simulink library "PhD_Library"  (R2018a)
settings: Solver=VariableStepAuto  StartTime=0.0  StopTime=10.0  RelTol=1e-3
values from neighbouring files (symbols this model uses):
  Ts = Ts_c    (= 1e-07)    [PlantStateEquations_abc_Script.m]
undefined symbols (not defined in the file or in its folder): D1, Delta, DiscIntNeverNeededParam, ESS, f_LPF_noise, fcutouti, fcutoutv, fn, fsw, Iap, Kp, PCC, Sn, tctrl, Ti, Ts_control, Ts_PWM, Uabp, Uanp, WT, X, zeta
libraries: $bdroot x84, powerlib_meascontrol x59, powerlib x56, peTransforms x32, cstblocks x2, simulink x2
(part 3 of 5)

== system PhD_Library/Offshore_Oil_and_Wind/LSC_LCL_Trafo_NoSwitching ==
  Open_Close_Breaker : Inport
  Vabcref : Inport  Port=2
  Bus Creator : BusCreator  Inputs=6
  Controlled Voltage Source : powerlib/Electrical Sources/Controlled Voltage Source  Initialize=on  Source_Type=AC  Amplitude=Uab*(2/3)^0.5  Phase=30  Frequency=fn  Measurements=None
  Controlled Voltage Source1 : powerlib/Electrical Sources/Controlled Voltage Source  Initialize=on  Source_Type=AC  Amplitude=Uab*(2/3)^0.5  Phase=30-120  Frequency=fn  Measurements=None
  Controlled Voltage Source2 : powerlib/Electrical Sources/Controlled Voltage Source  Initialize=on  Source_Type=AC  Amplitude=Uab*(2/3)^0.5  Phase=30+120  Frequency=fn  Measurements=None
  Demux2 : Demux  Outputs=3
  HV : powerlib/Measurements/Three-Phase V-I Measurement  VoltageMeasurement=phase-to-ground  SetLabelV=off  LabelV=vgrid  Vpu=off  VpuLL=off  CurrentMeasurement=yes  SetLabelI=off  LabelI=igrid  Ipu=off  Pbase=sn  Vbase=uab  OutputType=Complex  PhasorSimulation=off  PSBequivalent=0
  High Res Grounding : powerlib/Elements/Three-Phase Parallel RLC Load  LConnTagsString=A|B|C  Configuration=Y (grounded)  NominalVoltage=Uab  Vabc=[1e3 1e3 1e3]  Vabcp=[1e3 1e3 1e3]  NominalFrequency=fn  UnbalancedPower=off  ActivePower=0.001  InductivePower=0  CapacitivePower=0  Pabc=[10e3 9e3 11e3]  QLabc=[100 90 110]  QCabc=[100 90 110]  Pabcp=[10e3 9e3 11e3]  QLabcp=[100 90 110]  QCabcp=[100 90 110]  Measurements=None  LoadType=constant Z
  INV : powerlib/Measurements/Three-Phase V-I Measurement  VoltageMeasurement=phase-to-ground  SetLabelV=off  LabelV=vconv  Vpu=off  VpuLL=off  CurrentMeasurement=yes  SetLabelI=off  LabelI=iconv  Ipu=off  Pbase=sn  Vbase=uab  OutputType=Complex  PhasorSimulation=off  PSBequivalent=0
  LV : powerlib/Measurements/Three-Phase V-I Measurement  VoltageMeasurement=phase-to-ground  SetLabelV=off  LabelV=vgrid  Vpu=off  VpuLL=off  CurrentMeasurement=yes  SetLabelI=off  LabelI=igrid  Ipu=off  Pbase=sn  Vbase=uab  OutputType=Complex  PhasorSimulation=off  PSBequivalent=0
  La_DVR1 : powerlib/Elements/Series RLC Branch  LConnTagsString=__new0  RConnTagsString=__new0  BranchType=RL  Resistance=Rf1  Inductance=Lf1  SetiL0=off  InitialCurrent=0  Capacitance=1.0  Setx0=off  InitialVoltage=0  Measurements=None
  La_DVR2 : powerlib/Elements/Series RLC Branch  LConnTagsString=__new0  RConnTagsString=__new0  BranchType=RL  Resistance=Rf1  Inductance=Lf1  SetiL0=off  InitialCurrent=0  Capacitance=1.0  Setx0=off  InitialVoltage=0  Measurements=None
  La_DVR3 : powerlib/Elements/Series RLC Branch  LConnTagsString=__new0  RConnTagsString=__new0  BranchType=RL  Resistance=Rf1  Inductance=Lf1  SetiL0=off  InitialCurrent=0  Capacitance=1.0  Setx0=off  InitialVoltage=0  Measurements=None
  La_DVR4 : powerlib/Elements/Series RLC Branch  LConnTagsString=__new0  RConnTagsString=__new0  BranchType=RC  Resistance=Rc  Inductance=Lf1  SetiL0=off  InitialCurrent=0  Capacitance=Cf  Setx0=off  InitialVoltage=0  Measurements=None
  La_DVR5 : powerlib/Elements/Series RLC Branch  LConnTagsString=__new0  RConnTagsString=__new0  BranchType=RC  Resistance=Rc  Inductance=Lf1  SetiL0=off  InitialCurrent=0  Capacitance=Cf  Setx0=off  InitialVoltage=0  Measurements=None
  La_DVR6 : powerlib/Elements/Series RLC Branch  LConnTagsString=__new0  RConnTagsString=__new0  BranchType=RC  Resistance=Rc  Inductance=Lf1  SetiL0=off  InitialCurrent=0  Capacitance=Cf  Setx0=off  InitialVoltage=0  Measurements=None
  Three-Phase Transformer (Two Windings) : powerlib/Elements/Three-Phase Transformer (Two Windings)  Winding1Connection=Y  Winding2Connection=Delta (D1)  CoreType=Three-limb core (core-type)  SetSaturation=off  Hysteresis=off  DataFile='hysteresis'  SetInitialFlux=off  Measurements=None  UNITS=pu  NominalPower=[ Sn , fn ]  Winding1=[ Uhv_ab , rf2/2 , lf2/2 ]  Winding2=[ Uab , rf2/2 , lf2/2 ]  Rm=500  Lm=500  L0=0.5  Saturation=[ 0,0 ; 0.0024,1.2 ; 1.0,1.52 ]  InitialFluxes=[0 0 0]  MoreParameters=off  BreakLoop=off  DataType=off  TransfoNumber=1
  Three-Phase Breaker : powerlib/Elements/Three-Phase Breaker  InitialState=open  SwitchA=on  SwitchB=on  SwitchC=on  SwitchTimes="[1/60  5/60]"  External=on  BreakerResistance=0.01  SnubberResistance=1e6  SnubberCapacitance=inf  Measurements=None
  A : PMIOPort  Side=Right
  B : PMIOPort  Port=2  Side=Right
  C : PMIOPort  Port=3  Side=Right
  m : Outport
  wires:
  HV/2 -> Bus Creator/2  "HV_Iabc"
  LV/1 -> Bus Creator/3  "LV_Vabc"
  INV/1 -> Bus Creator/5  "INV_Vabc"
  INV/2 -> Bus Creator/6  "INV_Iabc"
  HV/1 -> Bus Creator/1  "HV_Vabc"
  LV/2 -> Bus Creator/4  "LV_Iabc"
  Bus Creator/1 -> m/1
  Open_Close_Breaker/1 -> Three-Phase Breaker/1
  Vabcref/1 -> Demux2/1
  Demux2/1 -> Controlled Voltage Source/1  "Va"
  Demux2/2 -> Controlled Voltage Source1/1  "Vb"
  Demux2/3 -> Controlled Voltage Source2/1  "Vc"
  connections:
  La_DVR1/LConn1 -- INV/RConn1
  LV/RConn1 -- Three-Phase Transformer (Two Windings)/RConn1 -- High Res Grounding/LConn1
  La_DVR1/RConn1 -- La_DVR4/RConn1 -- LV/LConn1
  Three-Phase Transformer (Two Windings)/LConn3 -- HV/LConn3
  Three-Phase Transformer (Two Windings)/RConn3 -- LV/RConn3 -- High Res Grounding/LConn3
  La_DVR2/RConn1 -- La_DVR5/RConn1 -- LV/LConn2
  Three-Phase Transformer (Two Windings)/LConn2 -- HV/LConn2
  Three-Phase Transformer (Two Windings)/RConn2 -- LV/RConn2 -- High Res Grounding/LConn2
  Three-Phase Transformer (Two Windings)/LConn1 -- HV/LConn1
  LV/LConn3 -- La_DVR3/RConn1 -- La_DVR6/RConn1
  La_DVR3/LConn1 -- INV/RConn3
  La_DVR5/LConn1 -- La_DVR6/LConn1 -- La_DVR4/LConn1
  La_DVR2/LConn1 -- INV/RConn2
  Three-Phase Breaker/LConn2 -- B/RConn1
  Three-Phase Breaker/RConn2 -- HV/RConn2
  HV/RConn3 -- Three-Phase Breaker/RConn3
  Three-Phase Breaker/LConn3 -- C/RConn1
  HV/RConn1 -- Three-Phase Breaker/RConn1
  Three-Phase Breaker/LConn1 -- A/RConn1
  Controlled Voltage Source2/LConn1 -- Controlled Voltage Source/LConn1 -- Controlled Voltage Source1/LConn1
  INV/LConn1 -- Controlled Voltage Source/RConn1
  Controlled Voltage Source1/RConn1 -- INV/LConn2
  Controlled Voltage Source2/RConn1 -- INV/LConn3

== system PhD_Library/Offshore_Oil_and_Wind/PI_Kg_Kp_Ti_AntiWindup ==
  note: PI: Kg (Kp + 1/sTi)
  error : Inport
  DisableP : Inport  Port=2
  Ihold : Inport  Port=3
  force_int : Inport  Port=4
  force_val : Inport  Port=5
  Add1 : Sum
  Add9 : Sum
  Constant : Constant  Value=PI_max
  Constant1 : Constant  Value=PI_min
  Constant8 : Constant  Value=0
  Gain1 : Gain  Gain=Kp
  Gain7 : Gain  Gain=Kg
  Gain9 : Gain  Gain=1/Ti
  NotEqual : RelationalOperator  Operator=~=  OutDataTypeStr=boolean  RndMeth=Simplest
  Product : Product
  Relay : Relay  OnSwitchValue=0.6  OffSwitchValue=0.4  OnOutputValue=0  OffOutputValue=1
  Saturation1 : Saturate  UpperLimit=PI_max  LowerLimit=PI_min
  Switch : Switch  Criteria=u2 > Threshold
  digital_integrator : $bdroot/Offshore_Oil_and_Wind/digital_integrator  Ts=Ts
  out : Outport
  Punlim : Outport  Port=2
  I : Outport  Port=3
  wires:
  NotEqual/1 -> [StopInt]
  Saturation1/1 -> out/1, NotEqual/2
  error/1 -> Gain7/1
  digital_integrator/1 -> I/1, Add9/2
  Add1/1 -> Switch/2
  Constant8/1 -> Switch/1
  Gain7/1 -> Gain1/1, Switch/3
  Switch/1 -> Gain9/1
  Add9/1 -> NotEqual/1, Saturation1/1
  Gain9/1 -> digital_integrator/1
  [StopInt] -> Add1/1
  Ihold/1 -> Add1/2
  Product/1 -> Punlim/1, Add9/1
  Gain1/1 -> Product/2
  DisableP/1 -> Relay/1
  Relay/1 -> Product/1
  force_val/1 -> digital_integrator/5
  force_int/1 -> digital_integrator/4
  Constant1/1 -> digital_integrator/3
  Constant/1 -> digital_integrator/2

== system PhD_Library/Offshore_Oil_and_Wind/PI_Kp_Ti_AntiWindup ==
  note: PI: Kp (s Ti + 1) / (s Ti)
  error : Inport
  Ihold : Inport  Port=2
  force_int : Inport  Port=3
  force_val : Inport  Port=4
  Add1 : Sum
  Add9 : Sum
  Constant : Constant  Value=PI_max
  Constant1 : Constant  Value=PI_min
  Constant8 : Constant  Value=0
  Gain7 : Gain  Gain=Kp
  Gain9 : Gain  Gain=1/Ti
  NotEqual : RelationalOperator  Operator=~=  OutDataTypeStr=boolean  RndMeth=Simplest
  Saturation1 : Saturate  UpperLimit=PI_max  LowerLimit=PI_min
  Switch : Switch  Criteria=u2 > Threshold
  digital_integrator : $bdroot/Offshore_Oil_and_Wind/digital_integrator  Ts=Ts
  out : Outport
  Punlim : Outport  Port=2
  I : Outport  Port=3
  wires:
  NotEqual/1 -> [StopInt]
  Saturation1/1 -> out/1, NotEqual/2
  error/1 -> Gain7/1
  digital_integrator/1 -> I/1, Add9/2
  Add1/1 -> Switch/2
  Constant8/1 -> Switch/1
  Gain7/1 -> Switch/3, Punlim/1, Add9/1
  Switch/1 -> Gain9/1
  Add9/1 -> NotEqual/1, Saturation1/1
  Gain9/1 -> digital_integrator/1
  [StopInt] -> Add1/1
  Ihold/1 -> Add1/2
  Constant1/1 -> digital_integrator/3
  force_int/1 -> digital_integrator/4
  force_val/1 -> digital_integrator/5
  Constant/1 -> digital_integrator/2

== system PhD_Library/Offshore_Oil_and_Wind/PLL ==
  vabc : Inport
  PLL (3ph) : powerlib_meascontrol/PLL/PLL (3ph)  Fmin=0.8*fn  Par_Init=[PLL_ini, fn]  ParK=[Kp_pll, Ki_pll, Kd_pll]  TcD=1e-4  MaxRateChangeFreq=fn/5  FilterCutOffFreq=fn/2  Ts=Ts  AGC=on
  Rate Transition1 : RateTransition  OutPortSampleTime=Ts
  Rtot_pu1 : Gain  Gain=-1  SaturateOnIntegerOverflow=on  OutDataTypeStr=Inherit: Same as input  ParamDataTypeStr=Inherit: Same as input
  Rtot_pu3 : Gain  Gain=1/fn  SaturateOnIntegerOverflow=on  OutDataTypeStr=Inherit: Same as input  ParamDataTypeStr=Inherit: Same as input
  f_pu : Outport
  wt : Outport  Port=2
  minus_wt : Outport  Port=3
  wires:
  Rtot_pu3/1 -> f_pu/1
  vabc/1 -> Rate Transition1/1
  Rate Transition1/1 -> PLL (3ph)/1
  PLL (3ph)/2 -> Rtot_pu1/1, wt/1
  PLL (3ph)/1 -> Rtot_pu3/1
  Rtot_pu1/1 -> minus_wt/1

== system PhD_Library/Offshore_Oil_and_Wind/PLL_pu ==
  vabc : Inport
  PLL (3ph) : powerlib_meascontrol/PLL/PLL (3ph)  Fmin=0.8*fn  Par_Init=[PLL_ini, fn]  ParK=[Kp_pll, Ki_pll, Kd_pll]  TcD=1e-4  MaxRateChangeFreq=fn/5  FilterCutOffFreq=fn/2  Ts=Ts  AGC=on
  Rate Transition1 : RateTransition  OutPortSampleTime=Ts
  Rtot_pu3 : Gain  Gain=1/fn  SaturateOnIntegerOverflow=on  OutDataTypeStr=Inherit: Same as input  ParamDataTypeStr=Inherit: Same as input
  wt : Outport
  f_pu : Outport  Port=2
  wires:
  Rtot_pu3/1 -> f_pu/1
  vabc/1 -> Rate Transition1/1
  Rate Transition1/1 -> PLL (3ph)/1
  PLL (3ph)/2 -> wt/1
  PLL (3ph)/1 -> Rtot_pu3/1

== system PhD_Library/Offshore_Oil_and_Wind/PWM_abc_negwt ==
  vdq_abc : Inport
  Enable_abc : Inport  Port=2
  vdq_abc_negwt : Inport  Port=3
  Enable_negwt : Inport  Port=4
  Udc : Inport  Port=5
  wt : Inport  Port=6
  Add : Sum
  Bus Creator : BusCreator  Inputs=4
  Constant1 : Constant  Value=0
  Constant10 : Constant  Value=Uabp
  Constant11 : Constant  Value=0
  Gain : Gain  Gain=Uabp/3^0.5
  Gain1 : Gain  Gain=-1
  Mux1 : Mux  Inputs=[2 1]
  Mux3 : Mux  Inputs=[2 1]
  Overmodulation : powerlib_meascontrol/Pulse & Signal Generators/Overmodulation  OverModType=Third harmonic
      settings: SourceProductName=Simscape Power Systems  SourceProductBaseCode=PS
  PWM Gen : powerlib_meascontrol/Pulse & Signal Generators/PWM Generator (2-Level)  ModulatorType=Three-phase bridge (6 pulses)  ModulatorMode=Unsynchronized  Fc=fsw  Pc=PWM_Ini_Phase  nF=27  MinMax="[ -1  1 ]"  SamplingTechnique=Asymmetrical regular (double edge)  ModulatingSignals=off  m=0.8  Freq=60  Phase=0  Ts=Ts  ShowCarrierOutport=off
      settings: SourceProductName=Simscape Power Systems
  Product1 : Product  Inputs=***
  Product8 : Product  Inputs=*/
  Product9 : Product  Inputs=***
  Rate Transition1 : RateTransition  OutPortSampleTime=Ts
  Rate Transition3 : RateTransition  OutPortSampleTime=Ts
  Rate Transition5 : RateTransition  OutPortSampleTime=Ts
  Relay : Relay  OnSwitchValue=0.6  OffSwitchValue=0.4
  Relay1 : Relay  OnSwitchValue=0.6  OffSwitchValue=0.4
  Saturation : Saturate  UpperLimit=10*Uabp  LowerLimit=0.001*Uabp
  Unit Delay2 : UnitDelay  InitialCondition=Uabp  SampleTime=Ts
  dq0 to abc : powerlib_meascontrol/Transformations/dq0 to abc  Alignment=90 degrees behind phase A axis
  dq0 to abc1 : powerlib_meascontrol/Transformations/dq0 to abc  Alignment=90 degrees behind phase A axis
  pulses : Outport
  Uabcref : Outport  Port=2
  m : Outport  Port=3
  wires:
  dq0 to abc1/1 -> Add/2
  Gain1/1 -> dq0 to abc1/2
  Product1/1 -> Bus Creator/2, dq0 to abc1/1  "vdq0_ref_scaled_NEG"
  vdq_abc_negwt/1 -> Rate Transition1/1
  Constant1/1 -> Mux1/2
  Mux1/1 -> Product1/1
  Product8/1 -> Product1/2, Product9/2
  Rate Transition1/1 -> Mux1/1
  Gain/1 -> Uabcref/1
  Bus Creator/1 -> m/1
  vdq_abc/1 -> Rate Transition3/1
  PWM Gen/1 -> pulses/1
  Udc/1 -> Unit Delay2/1
  Overmodulation/1 -> PWM Gen/1, Bus Creator/4  "uabc_ref"
  Constant10/1 -> Product8/1
  wt/1 -> Rate Transition5/1
  Rate Transition3/1 -> Mux3/1
  Mux3/1 -> Product9/1
  Unit Delay2/1 -> Saturation/1
  Product9/1 -> Bus Creator/1, dq0 to abc/1  "vdq0_ref_scaled_POS"
  Rate Transition5/1 -> dq0 to abc/2, Gain1/1
  Constant11/1 -> Mux3/2
  dq0 to abc/1 -> Add/1
  Enable_abc/1 -> Relay/1
  Relay/1 -> Product9/3
  Enable_negwt/1 -> Relay1/1
  Relay1/1 -> Product1/3
  Add/1 -> Bus Creator/3, Overmodulation/1, Gain/1  "uabc_ref_bef_3rd"
  Saturation/1 -> Product8/2

== system PhD_Library/Offshore_Oil_and_Wind/PWM_abc_negwt_acb ==
  vdq_abc : Inport
  Enable_abc : Inport  Port=2
  vdq_abc_negwt : Inport  Port=3
  Enable_negwt : Inport  Port=4
  vdq_acb : Inport  Port=5
  Enable_acb : Inport  Port=6
  Udc : Inport  Port=7
  wt : Inport  Port=8
  Add : Sum  Inputs=+++
  Constant1 : Constant  Value=0
  Constant10 : Constant  Value=Uabp
  Constant11 : Constant  Value=0
  Constant2 : Constant  Value=0
  Gain : Gain  Gain=2/3
  Gain1 : Gain  Gain=-1
  Mux1 : Mux  Inputs=[2 1]
  Mux2 : Mux  Inputs=[2 1]
  Mux3 : Mux  Inputs=[2 1]
  Overmodulation : powerlib_meascontrol/Pulse & Signal Generators/Overmodulation  OverModType=Third harmonic
      settings: SourceProductName=Simscape Power Systems  SourceProductBaseCode=PS
  PWM Gen : powerlib_meascontrol/Pulse & Signal Generators/PWM Generator (2-Level)  ModulatorType=Three-phase bridge (6 pulses)  ModulatorMode=Unsynchronized  Fc=fsw  Pc=PWM_Ini_Phase  nF=27  MinMax="[ -1  1 ]"  SamplingTechnique=Asymmetrical regular (double edge)  ModulatingSignals=off  m=0.8  Freq=60  Phase=0  Ts=Ts  ShowCarrierOutport=off
      settings: SourceProductName=Simscape Power Systems
  Product{1..6,9} (7 alike) : Product  Inputs=**
  Product8 : Product  Inputs=*/
  Rate Transition{1..3,5} (4 alike) : RateTransition  OutPortSampleTime=Ts
  Relay : Relay  OnSwitchValue=0.6  OffSwitchValue=0.4
  Relay1 : Relay  OnSwitchValue=0.6  OffSwitchValue=0.4
  Relay2 : Relay  OnSwitchValue=0.6  OffSwitchValue=0.4
  Saturation : Saturate  UpperLimit=10*Uabp  LowerLimit=0.001*Uabp
  Selector1 : Selector  InputPortWidth=3  IndexOptions=Index vector (dialog)  Indices=[1 3 2]  OutputSizes=1
  Unit Delay2 : UnitDelay  InitialCondition=Uabp  SampleTime=Ts
  dq0 to abc : powerlib_meascontrol/Transformations/dq0 to abc  Alignment=90 degrees behind phase A axis
  dq0 to abc1 : powerlib_meascontrol/Transformations/dq0 to abc  Alignment=90 degrees behind phase A axis
  dq0 to abc2 : powerlib_meascontrol/Transformations/dq0 to abc  Alignment=90 degrees behind phase A axis
  pulses : Outport
  Uabcref : Outport  Port=2
  uabcref : Outport  Port=3
  wires:
  dq0 to abc1/1 -> Product4/2  "abc_negwt"
  Gain1/1 -> dq0 to abc1/2
  Product1/1 -> dq0 to abc1/1  "vdq0_ref_scaled_negwt"
  vdq_abc_negwt/1 -> Rate Transition1/1
  Constant1/1 -> Mux1/2
  Mux1/1 -> Product1/1
  Rate Transition1/1 -> Mux1/1
  Product6/1 -> Uabcref/1
  vdq_abc/1 -> Rate Transition3/1
  PWM Gen/1 -> pulses/1
  Udc/1 -> Unit Delay2/1
  Overmodulation/1 -> uabcref/1, PWM Gen/1  "uabc_ref"
  Constant10/1 -> Product8/1
  wt/1 -> Rate Transition5/1
  Rate Transition3/1 -> Mux3/1
  Mux3/1 -> Product9/1
  Unit Delay2/1 -> Gain/1, Saturation/1
  Product9/1 -> dq0 to abc/1  "vdq0_ref_scaled_abc"
  Rate Transition5/1 -> dq0 to abc/2, dq0 to abc2/2, Gain1/1
  Constant11/1 -> Mux3/2
  dq0 to abc/1 -> Product3/1  "abc"
  Enable_abc/1 -> Relay/1
  Enable_negwt/1 -> Relay1/1
  Add/1 -> Product6/1, Overmodulation/1  "uabc_ref_bef_3rd"
  Saturation/1 -> Product8/2
  Product8/1 -> Product2/2, Product1/2, Product9/2
  Rate Transition2/1 -> Mux2/1
  vdq_acb/1 -> Rate Transition2/1
  Enable_acb/1 -> Relay2/1
  Mux2/1 -> Product2/1
  Constant2/1 -> Mux2/2
  Product2/1 -> dq0 to abc2/1  "vdq0_ref_scaled_acb"
  dq0 to abc2/1 -> Selector1/1
  Selector1/1 -> Product5/2  "acb"
  Relay/1 -> Product3/2
  Product3/1 -> Add/1
  Product4/1 -> Add/2
  Relay1/1 -> Product4/1
  Relay2/1 -> Product5/1
  Product5/1 -> Add/3
  Gain/1 -> Product6/2

== system PhD_Library/Offshore_Oil_and_Wind/PWM_single_dual ==
  vdq_single : Inport
  Enable_single : Inport  Port=2
  vdq_dual_pos : Inport  Port=3
  vdq_dual_neg : Inport  Port=4
  Enable_dual : Inport  Port=5
  Udc : Inport  Port=6
  wt : Inport  Port=7
  Add : Sum  Inputs=+++
  Constant1 : Constant  Value=0
  Constant10 : Constant  Value=Uabp
  Constant11 : Constant  Value=0
  Constant2 : Constant  Value=0
  Gain : Gain  Gain=2/3
  Mux1 : Mux  Inputs=[2 1]
  Mux2 : Mux  Inputs=[2 1]
  Mux3 : Mux  Inputs=[2 1]
  Overmodulation : powerlib_meascontrol/Pulse & Signal Generators/Overmodulation  OverModType=Third harmonic
      settings: SourceProductName=Simscape Power Systems  SourceProductBaseCode=PS
  PWM Gen : powerlib_meascontrol/Pulse & Signal Generators/PWM Generator (2-Level)  ModulatorType=Three-phase bridge (6 pulses)  ModulatorMode=Unsynchronized  Fc=fsw  Pc=PWM_Ini_Phase  nF=27  MinMax="[ -1  1 ]"  SamplingTechnique=Asymmetrical regular (double edge)  ModulatingSignals=off  m=0.8  Freq=60  Phase=0  Ts=Ts  ShowCarrierOutport=off
      settings: SourceProductName=Simscape Power Systems
  Product{1..6,9} (7 alike) : Product  Inputs=**
  Product8 : Product  Inputs=*/
  Rate Transition{1..3,5} (4 alike) : RateTransition  OutPortSampleTime=Ts
  Relay : Relay  OnSwitchValue=0.6  OffSwitchValue=0.4
  Relay1 : Relay  OnSwitchValue=0.6  OffSwitchValue=0.4
  Saturation : Saturate  UpperLimit=10*Uabp  LowerLimit=0.001*Uabp
  Selector1 : Selector  InputPortWidth=3  IndexOptions=Index vector (dialog)  Indices=[1 3 2]  OutputSizes=1
  Unit Delay2 : UnitDelay  InitialCondition=Uabp  SampleTime=Ts
  dq0 to abc : powerlib_meascontrol/Transformations/dq0 to abc  Alignment=90 degrees behind phase A axis
  dq0 to abc1 : powerlib_meascontrol/Transformations/dq0 to abc  Alignment=90 degrees behind phase A axis
  dq0 to abc2 : powerlib_meascontrol/Transformations/dq0 to abc  Alignment=90 degrees behind phase A axis
  pulses : Outport
  Uabcref : Outport  Port=2
  uabcref : Outport  Port=3
  wires:
  dq0 to abc1/1 -> Product4/2  "abc_ref_dual_pos"
  Rate Transition5/1 -> dq0 to abc/2, dq0 to abc1/2, dq0 to abc2/2
  Product1/1 -> dq0 to abc1/1  "vdq0_ref_scaled_dual_pos"
  vdq_dual_pos/1 -> Rate Transition1/1
  Constant1/1 -> Mux1/2
  Mux1/1 -> Product1/1
  Rate Transition1/1 -> Mux1/1
  Product6/1 -> Uabcref/1
  vdq_single/1 -> Rate Transition3/1
  PWM Gen/1 -> pulses/1
  Udc/1 -> Unit Delay2/1
  Overmodulation/1 -> uabcref/1, PWM Gen/1  "uabc_ref"
  Constant10/1 -> Product8/1
  wt/1 -> Rate Transition5/1
  Rate Transition3/1 -> Mux3/1
  Mux3/1 -> Product9/1
  Unit Delay2/1 -> Gain/1, Saturation/1
  Product9/1 -> dq0 to abc/1  "vdq0_ref_scaled_single"
  Constant11/1 -> Mux3/2
  dq0 to abc/1 -> Product3/1  "abc_ref_single"
  Enable_single/1 -> Relay/1
  Enable_dual/1 -> Relay1/1
  Add/1 -> Product6/1, Overmodulation/1  "uabc_ref_bef_3rd"
  Saturation/1 -> Product8/2
  Product8/1 -> Product2/2, Product1/2, Product9/2
  Rate Transition2/1 -> Mux2/1
  vdq_dual_neg/1 -> Rate Transition2/1
  Mux2/1 -> Product2/1
  Constant2/1 -> Mux2/2
  Product2/1 -> dq0 to abc2/1  "vdq0_ref_scaled_dual_neg"
  dq0 to abc2/1 -> Selector1/1
  Selector1/1 -> Product5/2  "abc_ref_dual_neg"
  Relay/1 -> Product3/2
  Product3/1 -> Add/1
  Product4/1 -> Add/2
  Relay1/1 -> Product5/1, Product4/1
  Product5/1 -> Add/3
  Gain/1 -> Product6/2

== system PhD_Library/Offshore_Oil_and_Wind/SR_Rini_Sdom ==
  S : Inport
  R : Inport  Port=2
  MATLAB Function : MATLAB Function  TreatAsAtomicUnit=on  SystemSampleTime=Ts
      settings: RTWSystemCode=Inline
  Q : Outport
  Qbar : Outport  Port=2
  wires:
  S/1 -> MATLAB Function/1(S)
  MATLAB Function/1(Q) -> Q/1
  R/1 -> MATLAB Function/2(R)
  MATLAB Function/2(Qbar) -> Qbar/1

== system PhD_Library/Offshore_Oil_and_Wind/SR_Sini_Sdom ==
  S : Inport
  R : Inport  Port=2
  MATLAB Function : MATLAB Function  TreatAsAtomicUnit=on  SystemSampleTime=Ts
      settings: RTWSystemCode=Inline
  Q : Outport
  Qbar : Outport  Port=2
  wires:
  S/1 -> MATLAB Function/1(S)
  MATLAB Function/1(Q) -> Q/1
  R/1 -> MATLAB Function/2(R)
  MATLAB Function/2(Qbar) -> Qbar/1

== system PhD_Library/Offshore_Oil_and_Wind/Scaling_and_PWM ==
  vdq_ref_pos : Inport
  Udc : Inport  Port=2
  wt : Inport  Port=3
  vdq_ref_neg : Inport  Port=4
  Bus Creator : BusCreator  Inputs=3
  Constant1 : Constant  Value=0
  Constant10 : Constant  Value=Uabp
  Constant11 : Constant  Value=0
  Gain : Gain  Gain=Uabp/3^0.5
  Gain1 : Gain  Gain=-1
  Mux1 : Mux  Inputs=[2 1]
  Mux3 : Mux  Inputs=[2 1]
  Overmodulation : powerlib_meascontrol/Pulse & Signal Generators/Overmodulation  OverModType=Third harmonic
      settings: SourceProductName=Simscape Power Systems  SourceProductBaseCode=PS
  PWM Gen 1 : powerlib_meascontrol/Pulse & Signal Generators/PWM Generator (2-Level)  ModulatorType=Three-phase bridge (6 pulses)  ModulatorMode=Unsynchronized  Fc=fsw  Pc=PWM_Ini_Phase  nF=27  MinMax="[ -1  1 ]"  SamplingTechnique=Asymmetrical regular (double edge)  ModulatingSignals=off  m=0.8  Freq=60  Phase=0  Ts=Ts  ShowCarrierOutport=off
      settings: SourceProductName=Simscape Power Systems
  Product1 : Product  Inputs=**
  Product8 : Product  Inputs=*/
  Product9 : Product  Inputs=**
  Rate Transition1 : RateTransition  OutPortSampleTime=Ts
  Rate Transition3 : RateTransition  OutPortSampleTime=Ts
  Rate Transition5 : RateTransition  OutPortSampleTime=Ts
  Unit Delay2 : UnitDelay  SampleTime=Ts
  dq0 to abc : powerlib_meascontrol/Transformations/dq0 to abc  Alignment=90 degrees behind phase A axis
  dq0 to abc1 : powerlib_meascontrol/Transformations/dq0 to abc  Alignment=90 degrees behind phase A axis
  pulses : Outport
  Uabcref : Outport  Port=2
  m : Outport  Port=3
  uabc_ref_pos : Outport  Port=4
  uabc_ref_neg : Outport  Port=5
  wires:
  dq0 to abc/1 -> uabc_ref_pos/1, Gain/1, Bus Creator/2, Overmodulation/1  "uabc_ref_bef3rd"
  Constant11/1 -> Mux3/2
  Rate Transition5/1 -> Gain1/1, dq0 to abc/2
  Product9/1 -> Bus Creator/1, dq0 to abc/1  "Vdq0_ref_scaled"
  Unit Delay2/1 -> Product8/2
  Mux3/1 -> Product9/1
  Rate Transition3/1 -> Mux3/1
  wt/1 -> Rate Transition5/1
  Constant10/1 -> Product8/1
  Overmodulation/1 -> Bus Creator/3, PWM Gen 1/1  "uabc_ref"
  Udc/1 -> Unit Delay2/1
  PWM Gen 1/1 -> pulses/1
  vdq_ref_pos/1 -> Rate Transition3/1
  Bus Creator/1 -> m/1
  Gain/1 -> Uabcref/1
  Rate Transition1/1 -> Mux1/1
  Product8/1 -> Product1/2, Product9/2
  Mux1/1 -> Product1/1
  Constant1/1 -> Mux1/2
  vdq_ref_neg/1 -> Rate Transition1/1
  Product1/1 -> dq0 to abc1/1  "Vdq0_ref_scaled"
  Gain1/1 -> dq0 to abc1/2
  dq0 to abc1/1 -> uabc_ref_neg/1

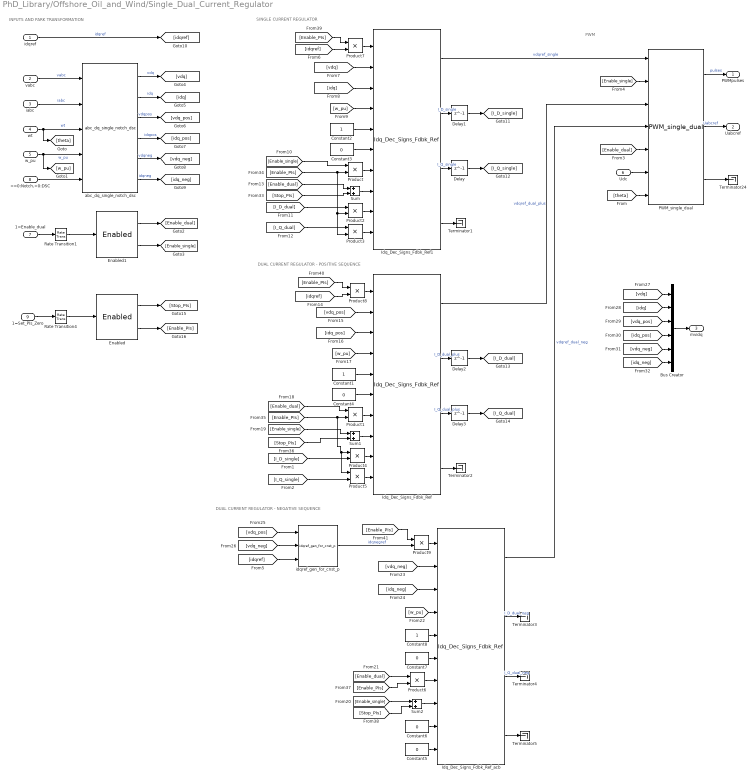
== system PhD_Library/Offshore_Oil_and_Wind/Single_Dual_Current_Regulator ==
  note: PWM
  note: DUAL CURRENT REGULATOR - NEGATIVE SEQUENCE
  note: DUAL CURRENT REGULATOR - POSITIVE SEQUENCE
  note: SINGLE CURRENT REGULATOR
  note: INPUTS AND PARK TRANSFORMATION
  idqref : Inport
  vabc : Inport  Port=2
  iabc : Inport  Port=3
  wt : Inport  Port=4
  w_pu : Inport  Port=5
  Udc : Inport  Port=6
  1=Enable_dual : Inport  Port=7
  <=0:Notch,>0:DSC : Inport  Port=8
  1=Set_PIs_Zero : Inport  Port=9
  Bus Creator : BusCreator  Inputs=6
  Constant1 : Constant
  Constant2 : Constant
  Constant{3..7} (5 alike) : Constant  Value=0
  Constant8 : Constant
  Delay{,1..3} (4 alike) : Delay  DelayLength=1  InitialCondition=0  SampleTime=Ts
  Enabled : $bdroot/Offshore_Oil_and_Wind/Enabled
  Enabled1 : $bdroot/Offshore_Oil_and_Wind/Enabled
  Idq_Dec_Signs_Fdbk_Ref : $bdroot/Offshore_Oil_and_Wind/Idq_Dec_Signs_Fdbk_Ref  Ts=Ts  fn=fgrid  Kp=PI_Kp  Ti=PI_Ti  L=PI_X  PI_max=PI_max  PI_min=PI_min  TrafoPhaseComp=0
  Idq_Dec_Signs_Fdbk_Ref1 : $bdroot/Offshore_Oil_and_Wind/Idq_Dec_Signs_Fdbk_Ref  Ts=Ts  fn=fgrid  Kp=PI_Kp  Ti=PI_Ti  L=PI_X  PI_max=PI_max  PI_min=PI_min  TrafoPhaseComp=0
  Idq_Dec_Signs_Fdbk_Ref_acb : $bdroot/Offshore_Oil_and_Wind/Idq_Dec_Signs_Fdbk_Ref  Ts=Ts  fn=fgrid  Kp=PI_Kp  Ti=PI_Ti  L=PI_X  PI_max=PI_max  PI_min=PI_min  TrafoPhaseComp=0
  PWM_single_dual : $bdroot/Offshore_Oil_and_Wind/PWM_single_dual  fsw=PWM_fsw  Ts=PWM_Ts  Uabp=PWM_Uabp  PWM_Ini_Phase=PWM_Ini
  Product{,1..9} (10 alike) : Product
  Rate Transition1 : RateTransition  OutPortSampleTime=Ts
  Rate Transition4 : RateTransition  InitialCondition=1  OutPortSampleTime=Ts
  Sum : Sum
  Sum1 : Sum
  Sum2 : Sum
  Terminator{1..5,24} (6 alike) : Terminator
  abc_dq_single_notch_dsc : $bdroot/Offshore_Oil_and_Wind/abc_dq_single_notch_dsc  Ts=Ts  fn=2*fgrid  zeta=zetanotch
  idqref_gen_for_cnst_p : $bdroot/Offshore_Oil_and_Wind/idqref_gen_for_cnst_p  Ts_control=Ts
  PWMpulses : Outport
  Uabcref : Outport  Port=2
  mvidq : Outport  Port=3
  wires:
  Udc/1 -> PWM_single_dual/6
  PWM_single_dual/3 -> Terminator24/1
  PWM_single_dual/2 -> Uabcref/1  "Uabcref"
  [idqref] -> idqref_gen_for_cnst_p/3
  [theta] -> PWM_single_dual/7
  PWM_single_dual/1 -> PWMpulses/1  "pulses"
  [Enable_dual] -> PWM_single_dual/5
  [Enable_single] -> PWM_single_dual/2
  vabc/1 -> abc_dq_single_notch_dsc/1  "vabc"
  iabc/1 -> abc_dq_single_notch_dsc/2  "iabc"
  wt/1 -> [theta], abc_dq_single_notch_dsc/3  "wt"
  w_pu/1 -> abc_dq_single_notch_dsc/4, [w_pu]  "w_pu"
  abc_dq_single_notch_dsc/1 -> [vdq]  "vdq"
  abc_dq_single_notch_dsc/2 -> [idq]  "idq"
  abc_dq_single_notch_dsc/3 -> [vdq_pos]  "vdqpos"
  abc_dq_single_notch_dsc/4 -> [idq_pos]  "idqpos"
  abc_dq_single_notch_dsc/5 -> [vdq_neg]  "vdqneg"
  abc_dq_single_notch_dsc/6 -> [idq_neg]  "idqneg"
  idqref/1 -> [idqref]  "idqref"
  [idqref] -> Product7/2
  [vdq] -> Idq_Dec_Signs_Fdbk_Ref1/2
  [idq] -> Idq_Dec_Signs_Fdbk_Ref1/3
  [w_pu] -> Idq_Dec_Signs_Fdbk_Ref1/4
  Constant2/1 -> Idq_Dec_Signs_Fdbk_Ref1/5
  Constant3/1 -> Idq_Dec_Signs_Fdbk_Ref1/6
  <=0:Notch,>0:DSC/1 -> abc_dq_single_notch_dsc/5
  [Enable_single] -> Product/1
  Idq_Dec_Signs_Fdbk_Ref1/3 -> Delay/1  "I_Q_single"
  Idq_Dec_Signs_Fdbk_Ref1/2 -> Delay1/1  "I_D_single"
  Idq_Dec_Signs_Fdbk_Ref/2 -> Delay2/1  "I_D_dual_plus"
  Idq_Dec_Signs_Fdbk_Ref/3 -> Delay3/1  "I_Q_dual_plus"
  Delay1/1 -> [I_D_single]
  Delay/1 -> [I_Q_single]
  Delay2/1 -> [I_D_dual]
  Delay3/1 -> [I_Q_dual]
  [I_D_single] -> Product4/2
  [I_Q_single] -> Product5/2
  [I_D_dual] -> Product2/1
  [I_Q_dual] -> Product3/1
  [Enable_dual] -> Sum/1
  [idqref] -> Product8/2
  [vdq_pos] -> Idq_Dec_Signs_Fdbk_Ref/2
  [idq_pos] -> Idq_Dec_Signs_Fdbk_Ref/3
  [w_pu] -> Idq_Dec_Signs_Fdbk_Ref/4
  Constant1/1 -> Idq_Dec_Signs_Fdbk_Ref/5
  Constant4/1 -> Idq_Dec_Signs_Fdbk_Ref/6
  [Enable_dual] -> Product1/1
  [Enable_single] -> Sum1/1
  Idq_Dec_Signs_Fdbk_Ref1/4 -> Terminator1/1
  Idq_Dec_Signs_Fdbk_Ref/4 -> Terminator2/1
  Idq_Dec_Signs_Fdbk_Ref_acb/2 -> Terminator3/1  "I_D_dual_neg"
  Idq_Dec_Signs_Fdbk_Ref_acb/3 -> Terminator4/1  "I_Q_dual_neg"
  Idq_Dec_Signs_Fdbk_Ref_acb/4 -> Terminator5/1
  Constant5/1 -> Idq_Dec_Signs_Fdbk_Ref_acb/10
  Constant6/1 -> Idq_Dec_Signs_Fdbk_Ref_acb/9
  [Enable_single] -> Sum2/1
  [Enable_dual] -> Product6/1
  Constant7/1 -> Idq_Dec_Signs_Fdbk_Ref_acb/6
  Constant8/1 -> Idq_Dec_Signs_Fdbk_Ref_acb/5
  [w_pu] -> Idq_Dec_Signs_Fdbk_Ref_acb/4
  [vdq_neg] -> Idq_Dec_Signs_Fdbk_Ref_acb/2
  [idq_neg] -> Idq_Dec_Signs_Fdbk_Ref_acb/3
  [vdq_pos] -> idqref_gen_for_cnst_p/1
  [vdq_neg] -> idqref_gen_for_cnst_p/2
  idqref_gen_for_cnst_p/1 -> Product9/2  "idqnegref"
  Idq_Dec_Signs_Fdbk_Ref1/1 -> PWM_single_dual/1  "vdqref_single"
  Idq_Dec_Signs_Fdbk_Ref/1 -> PWM_single_dual/3  "vdqref_dual_plus"
  Idq_Dec_Signs_Fdbk_Ref_acb/1 -> PWM_single_dual/4  "vdqref_dual_neg"
  Bus Creator/1 -> mvidq/1
  [vdq] -> Bus Creator/1
  [idq] -> Bus Creator/2
  [vdq_pos] -> Bus Creator/3
  [idq_pos] -> Bus Creator/4
  [vdq_neg] -> Bus Creator/5
  [idq_neg] -> Bus Creator/6
  1=Set_PIs_Zero/1 -> Rate Transition4/1
  Enabled/1 -> [Stop_PIs]
  Enabled/2 -> [Enable_PIs]
  [Enable_PIs] -> Product3/2, Product2/2, Product/2
  Product/1 -> Idq_Dec_Signs_Fdbk_Ref1/7
  Sum/1 -> Idq_Dec_Signs_Fdbk_Ref1/8
  Product3/1 -> Idq_Dec_Signs_Fdbk_Ref1/10
  [Stop_PIs] -> Sum/2
  Product2/1 -> Idq_Dec_Signs_Fdbk_Ref1/9
  Product1/1 -> Idq_Dec_Signs_Fdbk_Ref/7
  [Enable_PIs] -> Product5/1, Product4/1, Product1/2
  Sum1/1 -> Idq_Dec_Signs_Fdbk_Ref/8
  [Stop_PIs] -> Sum1/2
  Product5/1 -> Idq_Dec_Signs_Fdbk_Ref/10
  Product4/1 -> Idq_Dec_Signs_Fdbk_Ref/9
  [Enable_PIs] -> Product6/2
  Product6/1 -> Idq_Dec_Signs_Fdbk_Ref_acb/7
  [Stop_PIs] -> Sum2/2
  Sum2/1 -> Idq_Dec_Signs_Fdbk_Ref_acb/8
  [Enable_PIs] -> Product7/1
  Product7/1 -> Idq_Dec_Signs_Fdbk_Ref1/1
  [Enable_PIs] -> Product8/1
  Product8/1 -> Idq_Dec_Signs_Fdbk_Ref/1
  [Enable_PIs] -> Product9/1
  Product9/1 -> Idq_Dec_Signs_Fdbk_Ref_acb/1
  Rate Transition4/1 -> Enabled/1
  Enabled1/1 -> [Enable_dual]
  Enabled1/2 -> [Enable_single]
  Rate Transition1/1 -> Enabled1/1
  1=Enable_dual/1 -> Rate Transition1/1

== system PhD_Library/Offshore_Oil_and_Wind/Storage ==
  x : Inport
  Store if>0 : Inport  Port=2
  MATLAB Function : MATLAB Function  SystemSampleTime=Ts
      settings: RTWSystemCode=Inline
  y : Outport
  wires:
  MATLAB Function/1(y) -> y/1
  x/1 -> MATLAB Function/1(x)
  Store if>0/1 -> MATLAB Function/2(store)

== system PhD_Library/Offshore_Oil_and_Wind/Uac_Controller ==
  vac_setpoint : Inport
  vac : Inport  Port=2
  Ihold : Inport  Port=3
  DisableP : Inport  Port=4
  pre_mult_error : Inport  Port=5
  force_int : Inport  Port=6
  force_val : Inport  Port=7
  PI_Kg_Kp_Ti_AntiWindup : $bdroot/Offshore_Oil_and_Wind/PI_Kg_Kp_Ti_AntiWindup  Ts=Ts  Kg=Kg  Kp=Kp  Ti=Ti  PI_max=PI_max  PI_min=PI_min
  Product : Product
  Rate Transition1 : RateTransition  InitialCondition=1  OutPortSampleTime=Ts
  Rate Transition2 : RateTransition  InitialCondition=1  OutPortSampleTime=Ts
  Rate Transition3 : RateTransition  OutPortSampleTime=Ts
  Subtract : Sum  Inputs=+-
  Terminator2 : Terminator
  Terminator3 : Terminator
  iqref : Outport
  wires:
  PI_Kg_Kp_Ti_AntiWindup/2 -> Terminator2/1
  vac/1 -> Rate Transition1/1  "vac"
  PI_Kg_Kp_Ti_AntiWindup/3 -> Terminator3/1
  Subtract/1 -> Product/2
  Rate Transition1/1 -> Subtract/1
  Rate Transition2/1 -> Subtract/2
  PI_Kg_Kp_Ti_AntiWindup/1 -> iqref/1  "Idref"
  Ihold/1 -> PI_Kg_Kp_Ti_AntiWindup/3
  vac_setpoint/1 -> Rate Transition2/1
  DisableP/1 -> PI_Kg_Kp_Ti_AntiWindup/2
  force_val/1 -> PI_Kg_Kp_Ti_AntiWindup/5
  force_int/1 -> PI_Kg_Kp_Ti_AntiWindup/4
  pre_mult_error/1 -> Rate Transition3/1
  Rate Transition3/1 -> Product/1
  Product/1 -> PI_Kg_Kp_Ti_AntiWindup/1

== system PhD_Library/Offshore_Oil_and_Wind/Udc_Controller ==
  vdc : Inport
  Ihold : Inport  Port=2
  pre_mult_error : Inport  Port=3
  force_int : Inport  Port=4
  force_val : Inport  Port=5
  Constant1 : Constant
  PI_Kp_Ti_AntiWindup : $bdroot/Offshore_Oil_and_Wind/PI_Kp_Ti_AntiWindup  Ts=Ts  Kp=Kp  Ti=Ti  PI_max=PI_max  PI_min=PI_min
  Product : Product
  Rate Transition1 : RateTransition  InitialCondition=1  OutPortSampleTime=Ts
  Rate Transition3 : RateTransition  OutPortSampleTime=Ts
  Subtract : Sum  Inputs=+-
  Terminator2 : Terminator
  Terminator3 : Terminator
  idref : Outport
  wires:
  PI_Kp_Ti_AntiWindup/2 -> Terminator2/1
  vdc/1 -> Rate Transition1/1  "vdc"
  PI_Kp_Ti_AntiWindup/3 -> Terminator3/1
  Subtract/1 -> Product/2
  Rate Transition1/1 -> Subtract/1
  Constant1/1 -> Subtract/2
  PI_Kp_Ti_AntiWindup/1 -> idref/1  "Idref"
  Ihold/1 -> PI_Kp_Ti_AntiWindup/2
  Rate Transition3/1 -> Product/1
  pre_mult_error/1 -> Rate Transition3/1
  Product/1 -> PI_Kp_Ti_AntiWindup/1
  force_int/1 -> PI_Kp_Ti_AntiWindup/3
  force_val/1 -> PI_Kp_Ti_AntiWindup/4

== system PhD_Library/Offshore_Oil_and_Wind/abc-dq_DDSRF_PLL_Based ==
  Vabc : Inport
  wt : Inport  Port=2
  Iabc : Inport  Port=3
  Digital first order LPF{1..4} (4 alike) : $bdroot/Offshore_Oil_and_Wind/Digital first order LPF  Ts=Ts  fcutout=fc
  Inverse Park Transform{,1..3} (4 alike) : peTransforms/Inverse Park Transform  AxisAlignment=Q-axis  PowerInvariant=off
  Park Transform{,1..7} (8 alike) : peTransforms/Park Transform  AxisAlignment=Q-axis  PowerInvariant=off
  Rate Transition1 : RateTransition  OutPortSampleTime=Ts
  Rate Transition2 : RateTransition  OutPortSampleTime=Ts
  Rate Transition3 : RateTransition  OutPortSampleTime=Ts
  Selector : Selector  InputPortWidth=3  IndexOptions=Index vector (dialog)  Indices=2  OutputSizes=1
  Selector{9..12} (4 alike) : Selector  InputPortWidth=3  IndexOptions=Index vector (dialog)  Indices=[1 2]  OutputSizes=1
  Selector{2..4,6..8} (6 alike) : Selector  InputPortWidth=3  IndexOptions=Index vector (dialog)  Indices=[1 3 2]  OutputSizes=1
  Subtract : Sum  Inputs=+-
  Subtract1 : Sum  Inputs=-+
  Subtract2 : Sum  Inputs=+-
  Subtract3 : Sum  Inputs=-+
  q+_forPLL : Outport
  vdq+ : Outport  Port=2
  vdq- : Outport  Port=3
  idq+ : Outport  Port=4
  idq- : Outport  Port=5
  wires:
  Selector/1 -> q+_forPLL/1  "q+_forPLL"
  [teta] -> Inverse Park Transform2/2, Inverse Park Transform3/2
  Rate Transition3/1 -> Selector8/1, Park Transform4/1
  Selector11/1 -> vdq-/1
  Rate Transition1/1 -> Selector7/1, Park Transform/1
  Digital first order LPF4/1 -> Inverse Park Transform3/1, Selector10/1  "dq-"
  Inverse Park Transform3/1 -> Selector6/1
  Rate Transition2/1 -> [teta], Park Transform1/2, Park Transform/2
  Selector4/1 -> Park Transform3/1
  Iabc/1 -> Rate Transition3/1
  [teta] -> Park Transform6/2, Park Transform7/2
  Subtract2/1 -> Digital first order LPF3/1
  Park Transform1/1 -> Subtract1/2
  Selector6/1 -> Park Transform7/1
  Selector8/1 -> Park Transform5/1
  Park Transform7/1 -> Subtract2/2
  Digital first order LPF2/1 -> Selector11/1, Inverse Park Transform1/1  "dq-"
  Selector9/1 -> vdq+/1
  Inverse Park Transform1/1 -> Selector4/1
  Inverse Park Transform2/1 -> Selector2/1
  [teta] -> Park Transform2/2, Park Transform3/2
  Selector10/1 -> idq-/1
  Park Transform2/1 -> Subtract1/1
  Selector2/1 -> Park Transform6/1
  Park Transform5/1 -> Subtract3/2
  Subtract3/1 -> Digital first order LPF4/1
  Subtract1/1 -> Digital first order LPF2/1
  Park Transform/1 -> Subtract/1
  Digital first order LPF3/1 -> Inverse Park Transform2/1, Selector12/1  "dq+"
  Selector12/1 -> idq+/1
  Selector3/1 -> Park Transform2/1
  wt/1 -> Rate Transition2/1
  Park Transform6/1 -> Subtract3/1
  [teta] -> Park Transform5/2, Park Transform4/2
  Park Transform4/1 -> Subtract2/1
  Subtract/1 -> Digital first order LPF1/1, Selector/1
  [teta] -> Inverse Park Transform/2, Inverse Park Transform1/2
  Digital first order LPF1/1 -> Selector9/1, Inverse Park Transform/1  "dq+"
  Vabc/1 -> Rate Transition1/1
  Selector7/1 -> Park Transform1/1
  Inverse Park Transform/1 -> Selector3/1
  Park Transform3/1 -> Subtract/2

== system PhD_Library/Offshore_Oil_and_Wind/abc_dq ==
  vabc : Inport
  iabc : Inport  Port=2
  wt : Inport  Port=3
  Bus Creator : BusCreator  Inputs=4
  Digital first order LPF : $bdroot/Offshore_Oil_and_Wind/Digital first order LPF  Ts=Ts  fcutout=fcutoutv
  Digital first order LPF1 : $bdroot/Offshore_Oil_and_Wind/Digital first order LPF  Ts=Ts  fcutout=fcutouti
  Rate Transition1 : RateTransition  OutPortSampleTime=Ts
  Rate Transition2 : RateTransition  OutPortSampleTime=Ts
  Rate Transition4 : RateTransition  OutPortSampleTime=Ts
  Second-Order Filter1 : powerlib_meascontrol/Filters/Second-Order Filter  FilterType=Bandstop (Notch)  Fo=fn  Zeta=zeta  Ts=Ts  Initialize=off  Vac_Init="[0,  0,  60]"  Vdc_Init=0  PlotResponse=off  FreqRange=[0, 1000, 0.1]
      settings: SourceProductName=Simscape Power Systems  SourceProductBaseCode=PS
  Second-Order Filter5 : powerlib_meascontrol/Filters/Second-Order Filter  FilterType=Bandstop (Notch)  Fo=fn  Zeta=zeta  Ts=Ts  Initialize=off  Vac_Init="[0,  0,  60]"  Vdc_Init=0  PlotResponse=off  FreqRange=[0, 1000, 0.1]
      settings: SourceProductName=Simscape Power Systems  SourceProductBaseCode=PS
  Selector4 : Selector  InputPortWidth=3  IndexOptions=Index vector (dialog)  Indices=[1 2]  OutputSizes=1
  Selector5 : Selector  InputPortWidth=3  IndexOptions=Index vector (dialog)  Indices=[1 2]  OutputSizes=1
  abc to dq0 : powerlib_meascontrol/Transformations/abc to dq0  Alignment=90 degrees behind phase A axis
  abc to dq1 : powerlib_meascontrol/Transformations/abc to dq0  Alignment=90 degrees behind phase A axis
  vdq : Outport
  idq : Outport  Port=2
  m : Outport  Port=3
  wires:
  abc to dq1/1 -> Selector4/1
  Selector5/1 -> Digital first order LPF/1, Bus Creator/1  "vdq_unfilt"
  Rate Transition1/1 -> abc to dq0/1
  Rate Transition2/1 -> abc to dq1/2, abc to dq0/2
  Selector4/1 -> Bus Creator/2, Digital first order LPF1/1  "idq_unfilt"
  Rate Transition4/1 -> abc to dq1/1
  abc to dq0/1 -> Selector5/1
  Bus Creator/1 -> m/1
  Second-Order Filter5/1 -> vdq/1, Bus Creator/3  "vdq"
  wt/1 -> Rate Transition2/1
  vabc/1 -> Rate Transition1/1
  iabc/1 -> Rate Transition4/1
  Digital first order LPF1/1 -> Second-Order Filter1/1  "idq"
  Digital first order LPF/1 -> Second-Order Filter5/1  "vdq"
  Second-Order Filter1/1 -> Bus Creator/4, idq/1  "idq"

== system PhD_Library/Offshore_Oil_and_Wind/abc_dq_Rodriguez ==
  vabc : Inport
  wt : Inport  Port=2
  iabc : Inport  Port=3
  Digital first order LPF{1..4} (4 alike) : $bdroot/Offshore_Oil_and_Wind/Digital first order LPF  Ts=Ts  fcutout=fcutout
  Inverse Park Transform{,1..3} (4 alike) : peTransforms/Inverse Park Transform  AxisAlignment=Q-axis  PowerInvariant=off
  Park Transform{,1..7} (8 alike) : peTransforms/Park Transform  AxisAlignment=Q-axis  PowerInvariant=off
  Rate Transition1 : RateTransition  OutPortSampleTime=Ts
  Rate Transition2 : RateTransition  OutPortSampleTime=Ts
  Rate Transition3 : RateTransition  OutPortSampleTime=Ts
  Selector : Selector  InputPortWidth=3  IndexOptions=Index vector (dialog)  Indices=2  OutputSizes=1
  Selector{1..6} (6 alike) : Selector  InputPortWidth=3  IndexOptions=Index vector (dialog)  Indices=[1 3 2]  OutputSizes=1
  Selector{7..10} (4 alike) : Selector  InputPortWidth=3  IndexOptions=Index vector (dialog)  Indices=[1 2]  OutputSizes=1
  Subtract : Sum  Inputs=+-
  Subtract1 : Sum  Inputs=-+
  Subtract2 : Sum  Inputs=+-
  Subtract3 : Sum  Inputs=-+
  vq+_forPLL : Outport
  vdq+ : Outport  Port=2
  vdq- : Outport  Port=3
  idq+ : Outport  Port=4
  idq- : Outport  Port=5
  wires:
  Selector/1 -> vq+_forPLL/1  "q+_forPLL"
  Subtract/1 -> Selector/1, Digital first order LPF1/1
  Rate Transition1/1 -> Park Transform/1, Selector5/1
  wt/1 -> Rate Transition2/1
  Park Transform2/1 -> Subtract1/1
  Digital first order LPF1/1 -> Inverse Park Transform/1, Selector7/1  "dq+"
  Rate Transition2/1 -> Park Transform/2, Park Transform1/2, [teta]
  Subtract1/1 -> Digital first order LPF2/1
  Digital first order LPF2/1 -> Inverse Park Transform1/1, Selector8/1  "dq-"
  Park Transform/1 -> Subtract/1
  Park Transform1/1 -> Subtract1/2
  vabc/1 -> Rate Transition1/1
  iabc/1 -> Rate Transition3/1
  [teta] -> Inverse Park Transform1/2, Inverse Park Transform/2
  [teta] -> Park Transform3/2, Park Transform2/2
  Park Transform3/1 -> Subtract/2
  Selector5/1 -> Park Transform1/1
  Inverse Park Transform/1 -> Selector2/1
  Selector2/1 -> Park Transform2/1
  Inverse Park Transform1/1 -> Selector3/1
  Selector3/1 -> Park Transform3/1
  Rate Transition3/1 -> Park Transform4/1, Selector6/1
  [teta] -> Inverse Park Transform3/2, Inverse Park Transform2/2
  Inverse Park Transform2/1 -> Selector1/1
  Inverse Park Transform3/1 -> Selector4/1
  [teta] -> Park Transform7/2, Park Transform6/2
  Park Transform5/1 -> Subtract3/2
  Digital first order LPF3/1 -> Selector9/1, Inverse Park Transform2/1  "dq+"
  Subtract3/1 -> Digital first order LPF4/1
  Selector6/1 -> Park Transform5/1
  [teta] -> Park Transform4/2, Park Transform5/2
  Subtract2/1 -> Digital first order LPF3/1
  Selector4/1 -> Park Transform7/1
  Park Transform7/1 -> Subtract2/2
  Digital first order LPF4/1 -> Selector10/1, Inverse Park Transform3/1  "dq-"
  Park Transform4/1 -> Subtract2/1
  Park Transform6/1 -> Subtract3/1
  Selector1/1 -> Park Transform6/1
  Selector7/1 -> vdq+/1
  Selector8/1 -> vdq-/1
  Selector9/1 -> idq+/1
  Selector10/1 -> idq-/1

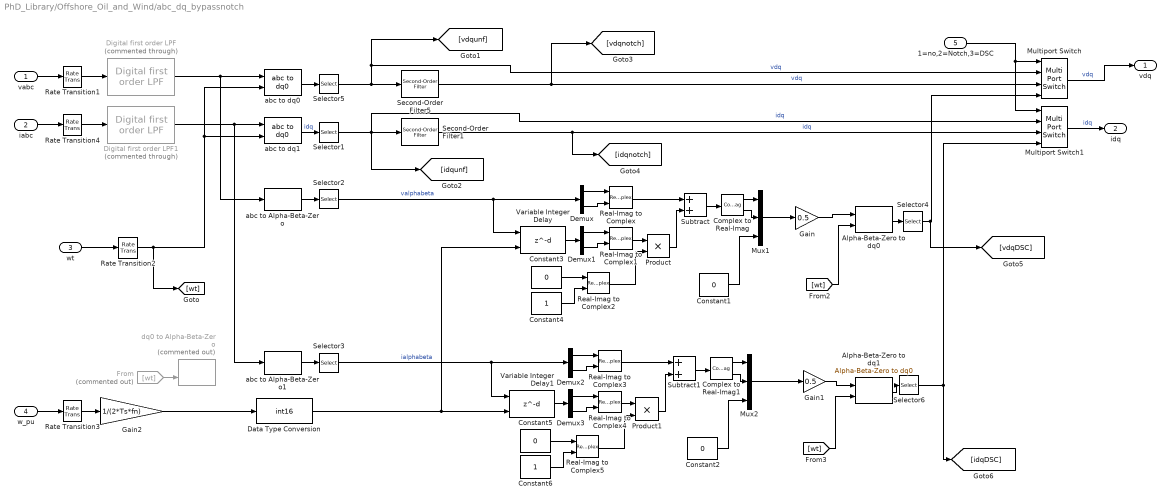
== system PhD_Library/Offshore_Oil_and_Wind/abc_dq_bypassnotch ==
  vabc : Inport
  iabc : Inport  Port=2
  wt : Inport  Port=3
  w_pu : Inport  Port=4
  1=no,2=Notch,3=DSC : Inport  Port=5
  Alpha-Beta-Zero to dq0 : powerlib_meascontrol/Transformations/Alpha-Beta-Zero to dq0  Alignment=90 degrees behind phase A axis
      settings: SourceProductName=Simscape Power Systems
  Alpha-Beta-Zero to dq1 : powerlib_meascontrol/Transformations/Alpha-Beta-Zero to dq0  Alignment=90 degrees behind phase A axis
      settings: SourceProductName=Simscape Power Systems
  Complex to Real-Imag : ComplexToRealImag
  Complex to Real-Imag1 : ComplexToRealImag
  Constant{1..3,5} (4 alike) : Constant  Value=0
  Constant4 : Constant
  Constant6 : Constant
  Data Type Conversion : DataTypeConversion  OutDataTypeStr=int16  RndMeth=Round  SaturateOnIntegerOverflow=on
  Demux{,1..3} (4 alike) : Demux  Outputs=2
  Digital first order LPF : $bdroot/Offshore_Oil_and_Wind/Digital first order LPF  Commented=through  Ts=Ts  fcutout=fcutoutv
  Digital first order LPF1 : $bdroot/Offshore_Oil_and_Wind/Digital first order LPF  Commented=through  Ts=Ts  fcutout=fcutouti
  From : From  Commented=on  GotoTag=wt
  Gain : Gain  Gain=0.5
  Gain1 : Gain  Gain=0.5
  Gain2 : Gain  Gain=1/(2*Ts*fn)
  Multiport Switch : MultiPortSwitch
  Multiport Switch1 : MultiPortSwitch
  Mux1 : Mux  Inputs=[1 1 1]
  Mux2 : Mux  Inputs=[1 1 1]
  Product : Product
  Product1 : Product
  Rate Transition1 : RateTransition  OutPortSampleTime=Ts
  Rate Transition2 : RateTransition  OutPortSampleTime=Ts
  Rate Transition3 : RateTransition  InitialCondition=1  OutPortSampleTime=Ts
  Rate Transition4 : RateTransition  OutPortSampleTime=Ts
  Real-Imag to Complex{,1..5} (6 alike) : RealImagToComplex
  Second-Order Filter1 : powerlib_meascontrol/Filters/Second-Order Filter  FilterType=Bandstop (Notch)  Fo=fn  Zeta=zeta  Ts=Ts  Initialize=off  Vac_Init="[0,  0,  60]"  Vdc_Init=0  PlotResponse=off  FreqRange=[0, 1000, 0.1]
      settings: SourceProductName=Simscape Power Systems  SourceProductBaseCode=PS
  Second-Order Filter5 : powerlib_meascontrol/Filters/Second-Order Filter  FilterType=Bandstop (Notch)  Fo=fn  Zeta=zeta  Ts=Ts  Initialize=off  Vac_Init="[0,  0,  60]"  Vdc_Init=0  PlotResponse=off  FreqRange=[0, 1000, 0.1]
      settings: SourceProductName=Simscape Power Systems  SourceProductBaseCode=PS
  Selector{1..6} (6 alike) : Selector  InputPortWidth=3  IndexOptions=Index vector (dialog)  Indices=[1 2]  OutputSizes=1
  Subtract : Sum
  Subtract1 : Sum
  Variable Integer Delay : Delay  DelayLengthSource=Input port  DelayLength=200  DelayLengthUpperLimit=500  SampleTime=Ts
      settings: InputPortMap=u0,p1
  Variable Integer Delay1 : Delay  DelayLengthSource=Input port  DelayLength=200  DelayLengthUpperLimit=500  SampleTime=Ts
      settings: InputPortMap=u0,p1
  abc to Alpha-Beta-Zero : powerlib_meascontrol/Transformations/abc to Alpha-Beta-Zero
      settings: SourceProductName=Simscape Power Systems
  abc to Alpha-Beta-Zero1 : powerlib_meascontrol/Transformations/abc to Alpha-Beta-Zero
      settings: SourceProductName=Simscape Power Systems
  abc to dq0 : powerlib_meascontrol/Transformations/abc to dq0  Alignment=90 degrees behind phase A axis
  abc to dq1 : powerlib_meascontrol/Transformations/abc to dq0  Alignment=90 degrees behind phase A axis
  dq0 to Alpha-Beta-Zero : powerlib_meascontrol/Transformations/dq0 to Alpha-Beta-Zero  Commented=on  Alignment=90 degrees behind phase A axis
      settings: SourceProductName=Simscape Power Systems  SourceProductBaseCode=PS
  vdq : Outport
  idq : Outport  Port=2
  wires:
  Rate Transition1/1 -> Digital first order LPF/1
  Rate Transition2/1 -> [wt], abc to dq1/2, abc to dq0/2
  Rate Transition4/1 -> Digital first order LPF1/1
  wt/1 -> Rate Transition2/1
  abc to dq1/1 -> Selector1/1  "idq"
  Selector5/1 -> Second-Order Filter5/1, [vdqunf], Multiport Switch/2  "vdq"
  Second-Order Filter5/1 -> [vdqnotch], Multiport Switch/3  "vdq"
  Second-Order Filter1/1 -> [idqnotch], Multiport Switch1/3  "idq"
  abc to dq0/1 -> Selector5/1
  Selector1/1 -> [idqunf], Second-Order Filter1/1, Multiport Switch1/2  "idq"
  abc to Alpha-Beta-Zero/1 -> Selector2/1
  abc to Alpha-Beta-Zero1/1 -> Selector3/1
  Gain2/1 -> Data Type Conversion/1
  From/1 -> dq0 to Alpha-Beta-Zero/2
  [wt] -> Alpha-Beta-Zero to dq0/2
  Alpha-Beta-Zero to dq0/1 -> Selector4/1
  Selector4/1 -> [vdqDSC], Multiport Switch/4
  Selector6/1 -> [idqDSC], Multiport Switch1/4
  [wt] -> Alpha-Beta-Zero to dq1/2
  Selector3/1 -> Demux2/1, Variable Integer Delay1/1  "ialphabeta"
  Alpha-Beta-Zero to dq1/1 -> Selector6/1
  Gain/1 -> Alpha-Beta-Zero to dq0/1
  Gain1/1 -> Alpha-Beta-Zero to dq1/1
  Variable Integer Delay/1 -> Demux1/1
  Constant1/1 -> Mux1/3
  Complex to Real-Imag/2 -> Mux1/2
  Constant4/1 -> Real-Imag to Complex2/2
  Complex to Real-Imag/1 -> Mux1/1
  Subtract/1 -> Complex to Real-Imag/1
  Real-Imag to Complex/1 -> Subtract/1
  Demux1/2 -> Real-Imag to Complex1/2
  Real-Imag to Complex1/1 -> Product/1
  Product/1 -> Subtract/2
  Real-Imag to Complex2/1 -> Product/2
  Constant3/1 -> Real-Imag to Complex2/1
  Demux1/1 -> Real-Imag to Complex1/1
  Demux/2 -> Real-Imag to Complex/2
  Demux/1 -> Real-Imag to Complex/1
  Selector2/1 -> Demux/1, Variable Integer Delay/1  "valphabeta"
  Mux1/1 -> Gain/1
  Mux2/1 -> Gain1/1
  Demux2/1 -> Real-Imag to Complex3/1
  Constant5/1 -> Real-Imag to Complex5/1
  Real-Imag to Complex5/1 -> Product1/2
  Demux3/1 -> Real-Imag to Complex4/1
  Product1/1 -> Subtract1/2
  Demux2/2 -> Real-Imag to Complex3/2
  Demux3/2 -> Real-Imag to Complex4/2
  Real-Imag to Complex3/1 -> Subtract1/1
  Constant6/1 -> Real-Imag to Complex5/2
  Real-Imag to Complex4/1 -> Product1/1
  Complex to Real-Imag1/1 -> Mux2/1
  Constant2/1 -> Mux2/3
  Complex to Real-Imag1/2 -> Mux2/2
  Variable Integer Delay1/1 -> Demux3/1
  Subtract1/1 -> Complex to Real-Imag1/1
  Digital first order LPF/1 -> abc to Alpha-Beta-Zero/1, abc to dq0/1
  Digital first order LPF1/1 -> abc to Alpha-Beta-Zero1/1, abc to dq1/1
  w_pu/1 -> Rate Transition3/1
  Rate Transition3/1 -> Gain2/1
  vabc/1 -> Rate Transition1/1
  iabc/1 -> Rate Transition4/1
  Data Type Conversion/1 -> Variable Integer Delay1/2, Variable Integer Delay/2
  Multiport Switch/1 -> vdq/1  "vdq"
  Multiport Switch1/1 -> idq/1  "idq"
  1=no,2=Notch,3=DSC/1 -> Multiport Switch1/1, Multiport Switch/1
